simulink model "Robust_RotPen"  (R2025b)
settings: Solver=VariableStepAuto  StartTime=0.0  StopTime=10  RelTol=1e-3
undefined symbols (not defined in the file or in its folder): K
libraries: cstblocks x1
settings Model: Creator=djangovanderplas  LastModifiedBy=djangovanderplas

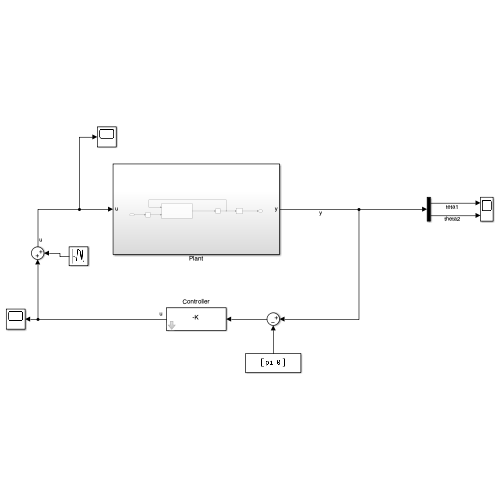
[thumbnail: Simulink's stored preview of the top-level diagram]
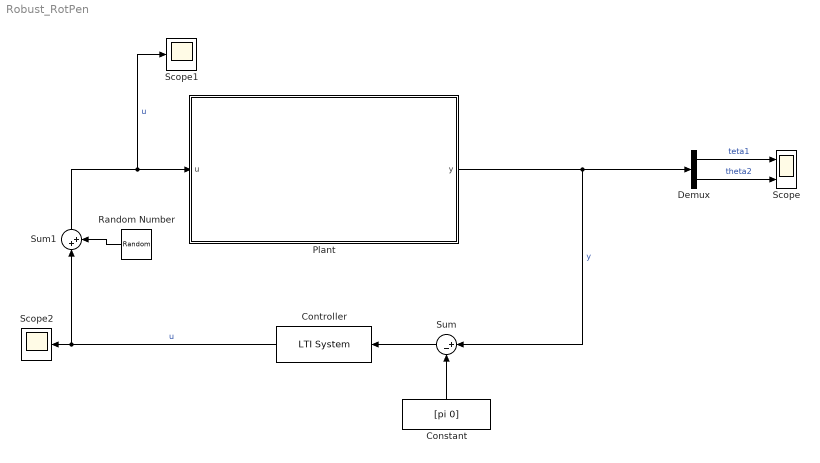
== system Robust_RotPen ==
  Constant : Constant  Value=[pi 0]
  Controller : cstblocks/LTI System  sys=-K  IC=[]  PadeOrder=0
  Demux : Demux  Outputs=2
  Plant : Subsystem
  Random Number : RandomNumber  Variance=0.01  SampleTime=0.01
  Scope : Scope  NumInputPorts=2
      settings: ActiveDisplayYMinimum=-0.58650694157432914  ActiveDisplayYMaximum=3.6669593999507506
  Scope1 : Scope
      settings: ActiveDisplayYMinimum=-20.074204638285423  ActiveDisplayYMaximum=15.432266857996424
  Scope2 : Scope
      settings: ActiveDisplayYMinimum=-1  ActiveDisplayYMaximum=1  DataLoggingVariableName=ScopeData2
  Sum : Sum  Inputs=|+-
  Sum1 : Sum  Inputs=|++
  wires:
  Plant/1(y) -> Sum/1, Demux/1  "y"
  Sum1/1 -> Plant/1(u), Scope1/1  "u"
  Sum/1 -> Controller/1
  Constant/1 -> Sum/2
  Controller/1 -> Sum1/1, Scope2/1  "u"
  Random Number/1 -> Sum1/2
  Demux/1 -> Scope/1  "teta1"
  Demux/2 -> Scope/2  "theta2"

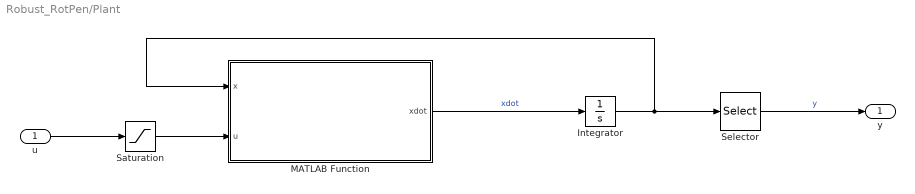
== system Robust_RotPen/Plant ==
  u : Inport
  Integrator : Integrator  InitialCondition=[pi+0.1;0;0;0]
  MATLAB Function : MATLAB Function  TreatAsAtomicUnit=on
  Saturation : Saturate  UpperLimit=1  LowerLimit=-1
  Selector : Selector  InputPortWidth=4  IndexOptions=Index vector (dialog)  Indices=[1 2]  OutputSizes=1
  y : Outport
  wires:
  u/1 -> Saturation/1
  Selector/1 -> y/1  "y"
  Integrator/1 -> Selector/1, MATLAB Function/1(x)
  MATLAB Function/1(xdot) -> Integrator/1  "xdot"
  Saturation/1 -> MATLAB Function/2(u)

== matlab function Robust_RotPen/Plant/MATLAB Function ==
  data: x input; u input; xdot output
function xdot = nonlinearPlant(x,u)

% State vector
theta1  = x(1);
theta2  = x(2);
dtheta1 = x(3);
dtheta2 = x(4);

% ============================================================
% Parameters
% ============================================================

pa       = 64.7915;
pb1      = 3.2117e3;
pc1      = 635.3865;
pg1      = 430.5226;
pu       = 2.2424e4;
p0       = 0;

pb2      = 0.0670;
pg2      = 112.0268;
pc2      = 0.2491;
psdelta2 = 0.1836;

epsv1    = 0.05;
epsv2    = 0.03;
vs2      = 3.5;

l1 = 0.1;
g  = 9.81;
pc = (l1/g)*pg2;

% ============================================================
% Dynamics
% ============================================================

c2 = cos(theta2);
s2 = sin(theta2);

% Inertia matrix
M11 = pa + 1 + 2*pc*c2;
M12 = 1 + pc*c2;
M21 = M12;
M22 = 1;

% Coriolis/Centrifugal terms
Cqdot1 = -pc*s2*(2*dtheta1*dtheta2 + dtheta2^2);
Cqdot2 =  pc*s2*dtheta1^2;

% Friction
F1 = pb1*dtheta1 + pc1*tanh(dtheta1/epsv1);

stribeck2 = pc2 + psdelta2*exp(-(dtheta2/vs2)^2);
F2 = pb2*dtheta2 + stribeck2*tanh(dtheta2/epsv2);

% Gravity
G1 = -pg1*sin(theta1) - pg2*sin(theta1 + theta2);
G2 = -pg2*sin(theta1 + theta2);

% Input torques
I1 = pu*u + p0;
I2 = 0;

% Right-hand side
rhs1 = I1 - Cqdot1 - F1 - G1;
rhs2 = I2 - Cqdot2 - F2 - G2;

% Solve M*qdd = rhs
detM = M11*M22 - M12*M21;

ddtheta1 = ( M22*rhs1 - M12*rhs2)/detM;
ddtheta2 = (-M21*rhs1 + M11*rhs2)/detM;

% State derivative
xdot = zeros(4,1);

xdot(1) = dtheta1;
xdot(2) = dtheta2;
xdot(3) = ddtheta1;
xdot(4) = ddtheta2;

end
